simulink model "chap7_2sim"  (R2019a)
settings: Solver=VariableStepAuto  StartTime=0.0  StopTime=5  RelTol=1e-3
settings Model: Creator=smilingfrog  LastModifiedBy=smilingfrog
settings DataIOCC: SaveOutput=off  SignalLogging=off  DSMLogging=off  SaveTime=off  ReturnWorkspaceOutputs=off

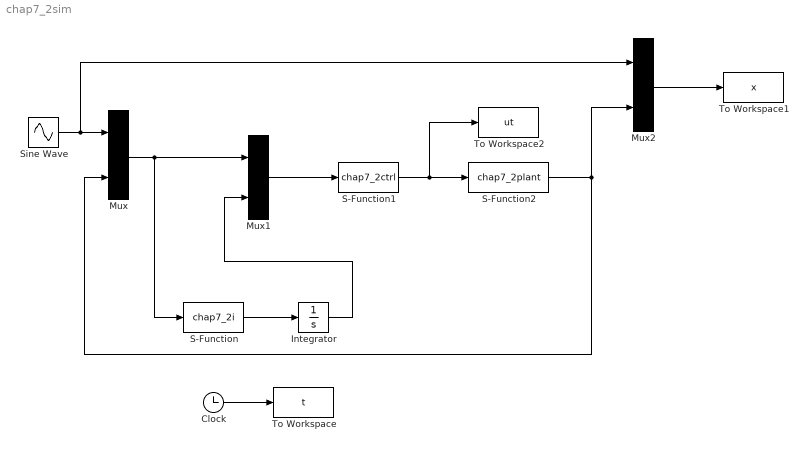
== system chap7_2sim ==
  Clock : Clock
  Integrator : Integrator
  Mux : Mux  Inputs=2
  Mux1 : Mux  Inputs=2
  Mux2 : Mux  Inputs=2
  S-Function : S-Function  FunctionName=chap7_2i  SFunctionDeploymentMode=off  EnableBusSupport=off
  S-Function1 : S-Function  FunctionName=chap7_2ctrl  SFunctionDeploymentMode=off  EnableBusSupport=off
  S-Function2 : S-Function  FunctionName=chap7_2plant  SFunctionDeploymentMode=off  EnableBusSupport=off
  Sine Wave : Sin  SampleTime=0
  To Workspace : ToWorkspace  VariableName=t  SampleTime=-1
  To Workspace1 : ToWorkspace  VariableName=x  SampleTime=-1
  To Workspace2 : ToWorkspace  VariableName=ut  SampleTime=-1
  wires:
  Sine Wave/1 -> Mux2/1, Mux/1
  Mux/1 -> S-Function/1, Mux1/1
  S-Function/1 -> Integrator/1
  Integrator/1 -> Mux1/2
  Mux1/1 -> S-Function1/1
  S-Function1/1 -> To Workspace2/1, S-Function2/1
  S-Function2/1 -> Mux/2, Mux2/2
  Clock/1 -> To Workspace/1
  Mux2/1 -> To Workspace1/1
